simulink model "M2_P1"  (R2023a)
settings: Solver=VariableStepAuto  StartTime=0.0  StopTime=500  RelTol=1e-3
values from neighbouring files (symbols this model uses):
  f_eff = 0.001    [varMotor.mat]    (also in varMotor2.mat = 0.022)
  J_eff = 4e-05    [varMotor.mat]    (also in varMotor2.mat = 0.00025)
  Kb = 0.02    [varMotor.mat]    (also in varMotor2.mat = 0.041)
  Ktn = 0.026    [varMotor.mat]    (also in varMotor2.mat = 0.047)
  L = 0.062    [varMotor.mat]    (also in varMotor2.mat)
  R = 2.5    [varMotor.mat]    (also in varMotor2.mat)
  time = 60    [varMotor.mat]    (also in varMotor2.mat)
settings Model: Creator=azzam  LastModifiedBy=azzam

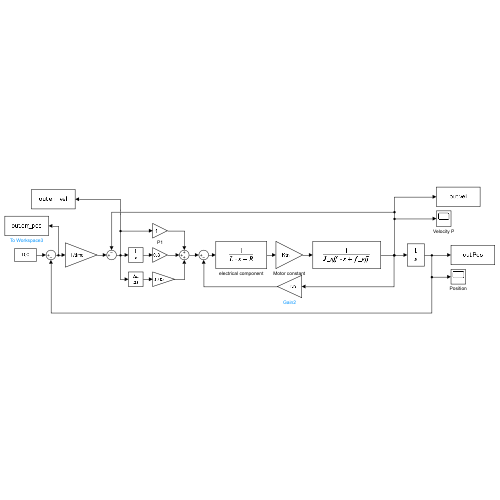
[thumbnail: Simulink's stored preview of the top-level diagram]
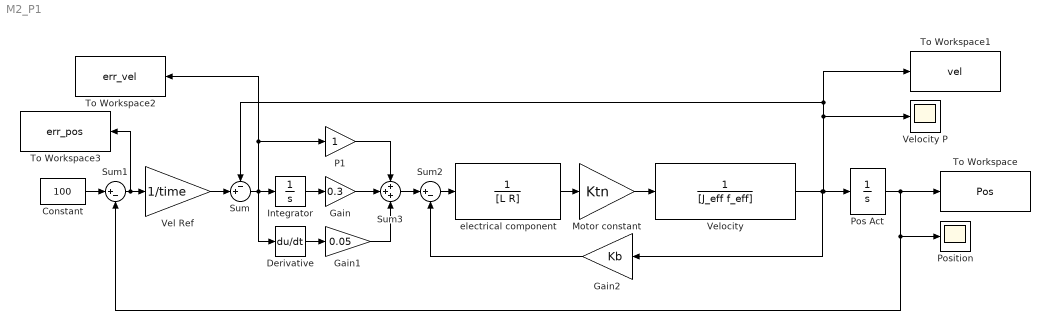
== system M2_P1 ==
  Constant : Constant  Value=100
  Derivative : Derivative
  Gain : Gain  Gain=0.3
  Gain1 : Gain  Gain=0.05
  Gain2 : Gain  Gain=Kb
  Integrator : Integrator
  Motor constant : Gain  Gain=Ktn
  P1 : Gain
  Pos Act : Integrator
  Position : Scope
  Sum : Sum  Inputs=-+|
  Sum1 : Sum  Inputs=|+-
  Sum2 : Sum  Inputs=|+-
  Sum3 : Sum  Inputs=+++
  To Workspace : ToWorkspace  VariableName=Pos  SaveFormat=Timeseries  SampleTime=-1
  To Workspace1 : ToWorkspace  VariableName=vel  SaveFormat=Timeseries  SampleTime=-1
  To Workspace2 : ToWorkspace  VariableName=err_vel  SaveFormat=Timeseries  SampleTime=-1
  To Workspace3 : ToWorkspace  VariableName=err_pos  SaveFormat=Timeseries  SampleTime=-1
  Vel Ref : Gain  Gain=1/time
  Velocity : TransferFcn  Denominator=[J_eff f_eff]
  Velocity P : Scope
  electrical component : TransferFcn  Denominator=[L R]
  wires:
  Sum1/1 -> To Workspace3/1, Vel Ref/1
  Vel Ref/1 -> Sum/2
  Velocity/1 -> To Workspace1/1, Sum/1, Velocity P/1, Pos Act/1, Gain2/1
  Constant/1 -> Sum1/1
  Gain2/1 -> Sum2/2
  Sum3/1 -> Sum2/1
  Sum2/1 -> electrical component/1
  Motor constant/1 -> Velocity/1
  electrical component/1 -> Motor constant/1
  P1/1 -> Sum3/1
  Gain1/1 -> Sum3/3
  Derivative/1 -> Gain1/1
  Gain/1 -> Sum3/2
  Integrator/1 -> Gain/1
  Sum/1 -> To Workspace2/1, P1/1, Derivative/1, Integrator/1
  Pos Act/1 -> To Workspace/1, Position/1, Sum1/2
